simulink model "EScooter_Physical_Architecture"  (R2025b)
settings: Solver=VariableStepAuto  StartTime=0.0  StopTime=10.0  RelTol=1e-3
settings Model: DataDictionary=EScooter_Interfaces.sldd  Creator=louis  LastModifiedBy=louis

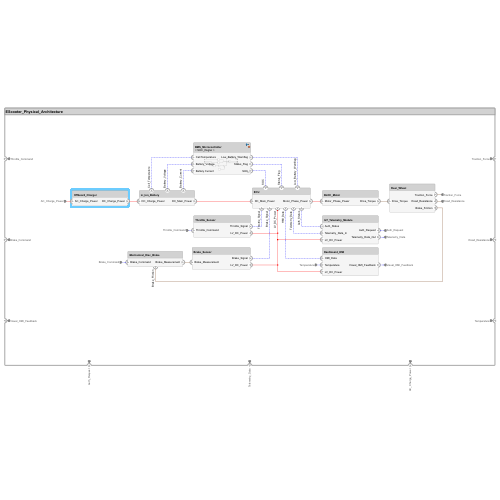
[thumbnail: Simulink's stored preview of the top-level diagram]
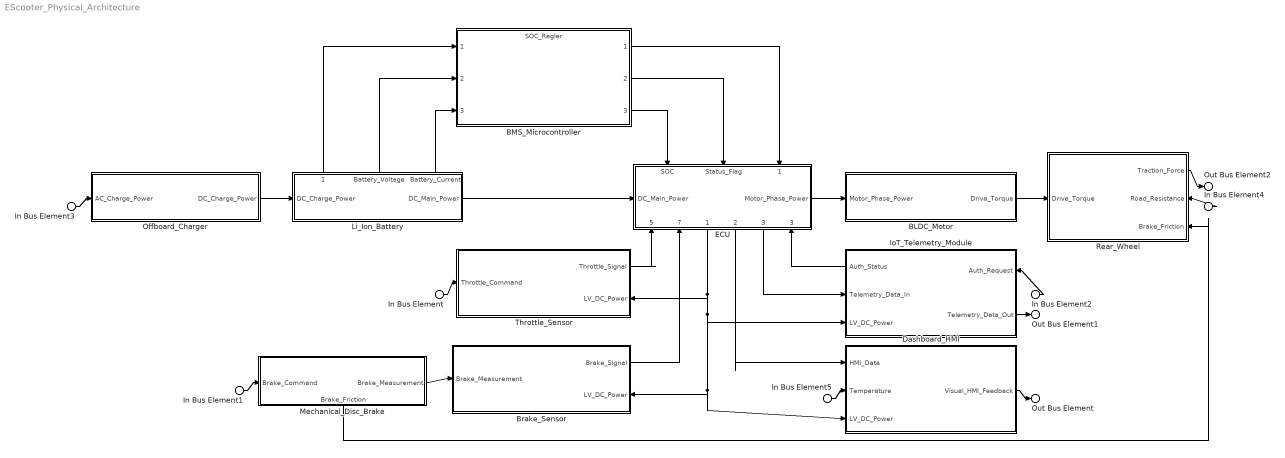
== system EScooter_Physical_Architecture ==
  In Bus Element : Inport  PortName=Throttle_Command
  In Bus Element1 : Inport  Port=2  PortName=Brake_Command
  In Bus Element2 : Inport  Port=3  PortName=Auth_Request
  In Bus Element3 : Inport  Port=4  PortName=AC_Charge_Power
  In Bus Element4 : Inport  Port=5  PortName=Road_Resistance
  In Bus Element5 : Inport  Port=6  PortName=Temperature
  BLDC_Motor : Subsystem
      settings: PortSchema="{\"entries\":[{\"content\":{\"headerSize\":26,\"margin\":15,\"minimumSpacing\":25,\"sides\":[{\"content\":{\"connectorIds\":[\"In1\"]},\"type\":\"ConnectorPlacement.EquallySpacedRectSide\",\"uuid\":\"c7864b0c-a654-4b38-88ce-65a12de73bec\"},{\"content\":{\"connectorIds\":[\"Out1\"],\"side\":\"RIGHT\"},\"type\":\"ConnectorPlacement.EquallySpacedRectSide\",\"uuid\":\"f08a465c-4605-4a04-9f25-0a3dbd0c3078\"},{\"content\":{\"side\":\"TOP\"},\"type\":\"ConnectorPlacement.EquallySpacedRectSide\",\"uuid\":\"8b4ebbb3-fc9a-4287-84ca-4c06f50a2e15\"}]},\"type\":\"ConnectorPlacement.EquallySpacedConnector\",\"uuid\":\"9d8a7b34-6d5f-451a-9c3e-baff170e8406\"}],\"packageUris\":[\"http://schema.mathworks.com/mf0/Connector/R2020b\"],\"version\":\"1.0\"}"
  BMS_Microcontroller : ModelReference  ModelNameDialog=SOC_Regler.slx  SimulationMode=Normal  ModelReferenceVersion=1.3
      settings: PortSchema="{\"entries\":[{\"content\":{\"headerSize\":38,\"margin\":15,\"minimumSpacing\":25,\"sides\":[{\"content\":{\"connectorIds\":[\"In1\",\"In2\",\"In3\"]},\"type\":\"ConnectorPlacement.EquallySpacedRectSide\",\"uuid\":\"4099fe1e-d8ea-4288-98e3-31b6343239af\"},{\"content\":{\"connectorIds\":[\"Out1\",\"Out2\",\"Out3\"],\"side\":\"RIGHT\"},\"type\":\"ConnectorPlacement.EquallySpacedRectSide\",\"uuid\":\"504c5db9-a45d-4379-96ce-ee806ba1f3a5\"},{\"content\":{\"side\":\"TOP\"},\"type\":\"ConnectorPlacement.EquallySpacedRectSide\",\"uuid\":\"29d2f34e-5430-431f-8925-f215a165c8d4\"}]},\"type\":\"ConnectorPlacement.EquallySpacedConnector\",\"uuid\":\"717a3a0c-5e38-4178-bc7e-8ddaf7311f91\"}],\"packageUris\":[\"http://schema.mathworks.com/mf0/Connector/R2020b\"],\"version\":\"1.0\"}"
  Brake_Sensor : Subsystem
      settings: PortSchema="{\"entries\":[{\"content\":{\"headerSize\":26,\"margin\":15,\"minimumSpacing\":25,\"sides\":[{\"content\":{\"connectorIds\":[\"In2\"]},\"type\":\"ConnectorPlacement.EquallySpacedRectSide\",\"uuid\":\"c7864b0c-a654-4b38-88ce-65a12de73bec\"},{\"content\":{\"connectorIds\":[\"Out1\",\"In1\"],\"side\":\"RIGHT\"},\"type\":\"ConnectorPlacement.EquallySpacedRectSide\",\"uuid\":\"f08a465c-4605-4a04-9f25-0a3dbd0c3078\"},{\"content\":{\"side\":\"TOP\"},\"type\":\"ConnectorPlacement.EquallySpacedRectSide\",\"uuid\":\"8b4ebbb3-fc9a-4287-84ca-4c06f50a2e15\"},{\"content\":{\"side\":\"BOTTOM\"},\"type\":\"ConnectorPlacement.EquallySpacedRectSide\",\"uuid\":\"60d35069-caa0-4e85-8360-19172966eb62\"}]},\"type\":\"ConnectorPlacement.EquallySpacedConnector\",\"uuid\":\"9d8a7b34-6d5f-451a-9c3e-baff170e8406\"}],\"packageUris\":[\"http://schema.mathworks.com/mf0/Connector/R2020b\"],\"version\":\"1.0\"}"
  Dashboard_HMI : Subsystem
      settings: PortSchema="{\"entries\":[{\"content\":{\"headerSize\":26,\"margin\":15,\"minimumSpacing\":25,\"sides\":[{\"content\":{\"connectorIds\":[\"In1\",\"In2\",\"In3\"]},\"type\":\"ConnectorPlacement.EquallySpacedRectSide\",\"uuid\":\"c7864b0c-a654-4b38-88ce-65a12de73bec\"},{\"content\":{\"connectorIds\":[\"Out1\"],\"side\":\"RIGHT\"},\"type\":\"ConnectorPlacement.EquallySpacedRectSide\",\"uuid\":\"f08a465c-4605-4a04-9f25-0a3dbd0c3078\"},{\"content\":{\"side\":\"TOP\"},\"type\":\"ConnectorPlacement.EquallySpacedRectSide\",\"uuid\":\"8b4ebbb3-fc9a-4287-84ca-4c06f50a2e15\"}]},\"type\":\"ConnectorPlacement.EquallySpacedConnector\",\"uuid\":\"9d8a7b34-6d5f-451a-9c3e-baff170e8406\"}],\"packageUris\":[\"http://schema.mathworks.com/mf0/Connector/R2020b\"],\"version\":\"1.0\"}"
  ECU : Subsystem
      settings: PortSchema="{\"entries\":[{\"content\":{\"headerSize\":26,\"margin\":15,\"minimumSpacing\":25,\"sides\":[{\"content\":{\"connectorIds\":[\"In6\"]},\"type\":\"ConnectorPlacement.EquallySpacedRectSide\",\"uuid\":\"c7864b0c-a654-4b38-88ce-65a12de73bec\"},{\"content\":{\"connectorIds\":[\"Out4\"],\"side\":\"RIGHT\"},\"type\":\"ConnectorPlacement.EquallySpacedRectSide\",\"uuid\":\"f08a465c-4605-4a04-9f25-0a3dbd0c3078\"},{\"content\":{\"connectorIds\":[\"In2\",\"In4\",\"In1\"],\"side\":\"TOP\"},\"type\":\"ConnectorPlacement.EquallySpacedRectSide\",\"uuid\":\"8b4ebbb3-fc9a-4287-84ca-4c06f50a2e15\"},{\"content\":{\"connectorIds\":[\"In5\",\"In7\",\"Out1\",\"Out2\",\"Out3\",\"In3\"],\"side\":\"BOTTOM\"},\"type\":\"ConnectorPlacement.EquallySpacedRectSide\",\"uuid\":\"c8544b79-1559-4f8f-8e3a-48f86e4e49c0\"}]},\"type\":\"ConnectorPlacement.EquallySpacedConnector\",\"uuid\":\"9d8a7b34-6d5f-451a-9c3e-baff170e8406\"}],\"packageUris\":[\"http://schema.mathworks.com/mf0/Connector/R2020b\"],\"version\":\"1.0\"}"
  IoT_Telemetry_Module : Subsystem
      settings: PortSchema="{\"entries\":[{\"content\":{\"headerSize\":26,\"margin\":15,\"minimumSpacing\":25,\"sides\":[{\"content\":{\"connectorIds\":[\"Out1\",\"In3\",\"In2\"]},\"type\":\"ConnectorPlacement.EquallySpacedRectSide\",\"uuid\":\"c7864b0c-a654-4b38-88ce-65a12de73bec\"},{\"content\":{\"connectorIds\":[\"In1\",\"Out2\"],\"side\":\"RIGHT\"},\"type\":\"ConnectorPlacement.EquallySpacedRectSide\",\"uuid\":\"f08a465c-4605-4a04-9f25-0a3dbd0c3078\"},{\"content\":{\"side\":\"TOP\"},\"type\":\"ConnectorPlacement.EquallySpacedRectSide\",\"uuid\":\"8b4ebbb3-fc9a-4287-84ca-4c06f50a2e15\"},{\"content\":{\"side\":\"BOTTOM\"},\"type\":\"ConnectorPlacement.EquallySpacedRectSide\",\"uuid\":\"026f311c-75bd-495b-b3f1-5519b50e0082\"}]},\"type\":\"ConnectorPlacement.EquallySpacedConnector\",\"uuid\":\"9d8a7b34-6d5f-451a-9c3e-baff170e8406\"}],\"packageUris\":[\"http://schema.mathworks.com/mf0/Connector/R2020b\"],\"version\":\"1.0\"}"
  Li_Ion_Battery : Subsystem
      settings: PortSchema="{\"entries\":[{\"content\":{\"headerSize\":26,\"margin\":15,\"minimumSpacing\":25,\"sides\":[{\"content\":{\"connectorIds\":[\"In1\"]},\"type\":\"ConnectorPlacement.EquallySpacedRectSide\",\"uuid\":\"c7864b0c-a654-4b38-88ce-65a12de73bec\"},{\"content\":{\"connectorIds\":[\"Out4\"],\"side\":\"RIGHT\"},\"type\":\"ConnectorPlacement.EquallySpacedRectSide\",\"uuid\":\"f08a465c-4605-4a04-9f25-0a3dbd0c3078\"},{\"content\":{\"connectorIds\":[\"Out1\",\"Out2\",\"Out3\"],\"side\":\"TOP\"},\"type\":\"ConnectorPlacement.EquallySpacedRectSide\",\"uuid\":\"8b4ebbb3-fc9a-4287-84ca-4c06f50a2e15\"},{\"content\":{\"side\":\"BOTTOM\"},\"type\":\"ConnectorPlacement.EquallySpacedRectSide\",\"uuid\":\"a12c9fad-78c1-47b3-951e-87e8443312d3\"}]},\"type\":\"ConnectorPlacement.EquallySpacedConnector\",\"uuid\":\"9d8a7b34-6d5f-451a-9c3e-baff170e8406\"}],\"packageUris\":[\"http://schema.mathworks.com/mf0/Connector/R2020b\"],\"version\":\"1.0\"}"
  Mechanical_Disc_Brake : Subsystem
      settings: PortSchema="{\"entries\":[{\"content\":{\"headerSize\":26,\"margin\":15,\"minimumSpacing\":25,\"sides\":[{\"content\":{\"connectorIds\":[\"In1\"]},\"type\":\"ConnectorPlacement.EquallySpacedRectSide\",\"uuid\":\"c0a0fd83-8e6b-4996-80ba-c62bfd1e5bac\"},{\"content\":{\"connectorIds\":[\"Out1\"],\"side\":\"RIGHT\"},\"type\":\"ConnectorPlacement.EquallySpacedRectSide\",\"uuid\":\"b459cc4e-9c94-4f14-9d9c-94419e22855a\"},{\"content\":{\"side\":\"TOP\"},\"type\":\"ConnectorPlacement.EquallySpacedRectSide\",\"uuid\":\"d2d10086-fe87-4682-8840-902f46fdf630\"},{\"content\":{\"connectorIds\":[\"Out2\"],\"side\":\"BOTTOM\"},\"type\":\"ConnectorPlacement.EquallySpacedRectSide\",\"uuid\":\"3ddfbb52-bdc8-43fc-9731-c09ce9f1a202\"}]},\"type\":\"ConnectorPlacement.EquallySpacedConnector\",\"uuid\":\"74f202a8-1c68-49b4-8447-64ee5fb276eb\"}],\"packageUris\":[\"http://schema.mathworks.com/mf0/Connector/R2020b\"],\"version\":\"1.0\"}"
  Offboard_Charger : Subsystem  Description=Ladeleistung 350W (Ausgeklammert aus SWaP, da nur im Charging-State aktiv)
      settings: PortSchema="{\"entries\":[{\"content\":{\"headerSize\":26,\"margin\":15,\"minimumSpacing\":25,\"sides\":[{\"content\":{\"connectorIds\":[\"In1\"]},\"type\":\"ConnectorPlacement.EquallySpacedRectSide\",\"uuid\":\"c0a0fd83-8e6b-4996-80ba-c62bfd1e5bac\"},{\"content\":{\"connectorIds\":[\"Out1\"],\"side\":\"RIGHT\"},\"type\":\"ConnectorPlacement.EquallySpacedRectSide\",\"uuid\":\"b459cc4e-9c94-4f14-9d9c-94419e22855a\"},{\"content\":{\"side\":\"TOP\"},\"type\":\"ConnectorPlacement.EquallySpacedRectSide\",\"uuid\":\"d2d10086-fe87-4682-8840-902f46fdf630\"}]},\"type\":\"ConnectorPlacement.EquallySpacedConnector\",\"uuid\":\"74f202a8-1c68-49b4-8447-64ee5fb276eb\"}],\"packageUris\":[\"http://schema.mathworks.com/mf0/Connector/R2020b\"],\"version\":\"1.0\"}"
  Rear_Wheel : Subsystem
      settings: PortSchema="{\"entries\":[{\"content\":{\"headerSize\":26,\"margin\":15,\"minimumSpacing\":25,\"sides\":[{\"content\":{\"connectorIds\":[\"In3\"]},\"type\":\"ConnectorPlacement.EquallySpacedRectSide\",\"uuid\":\"c7864b0c-a654-4b38-88ce-65a12de73bec\"},{\"content\":{\"connectorIds\":[\"Out1\",\"In1\",\"In2\"],\"side\":\"RIGHT\"},\"type\":\"ConnectorPlacement.EquallySpacedRectSide\",\"uuid\":\"f08a465c-4605-4a04-9f25-0a3dbd0c3078\"},{\"content\":{\"side\":\"TOP\"},\"type\":\"ConnectorPlacement.EquallySpacedRectSide\",\"uuid\":\"8b4ebbb3-fc9a-4287-84ca-4c06f50a2e15\"}]},\"type\":\"ConnectorPlacement.EquallySpacedConnector\",\"uuid\":\"9d8a7b34-6d5f-451a-9c3e-baff170e8406\"}],\"packageUris\":[\"http://schema.mathworks.com/mf0/Connector/R2020b\"],\"version\":\"1.0\"}"
  Throttle_Sensor : Subsystem
      settings: PortSchema="{\"entries\":[{\"content\":{\"headerSize\":26,\"margin\":15,\"minimumSpacing\":25,\"sides\":[{\"content\":{\"connectorIds\":[\"In2\"]},\"type\":\"ConnectorPlacement.EquallySpacedRectSide\",\"uuid\":\"c7864b0c-a654-4b38-88ce-65a12de73bec\"},{\"content\":{\"connectorIds\":[\"Out1\",\"In1\"],\"side\":\"RIGHT\"},\"type\":\"ConnectorPlacement.EquallySpacedRectSide\",\"uuid\":\"f08a465c-4605-4a04-9f25-0a3dbd0c3078\"},{\"content\":{\"side\":\"TOP\"},\"type\":\"ConnectorPlacement.EquallySpacedRectSide\",\"uuid\":\"8b4ebbb3-fc9a-4287-84ca-4c06f50a2e15\"}]},\"type\":\"ConnectorPlacement.EquallySpacedConnector\",\"uuid\":\"9d8a7b34-6d5f-451a-9c3e-baff170e8406\"}],\"packageUris\":[\"http://schema.mathworks.com/mf0/Connector/R2020b\"],\"version\":\"1.0\"}"
  Out Bus Element : Outport  PortName=Visual_HMI_Feedback
  Out Bus Element1 : Outport  Port=2  PortName=Telemetry_Data
  Out Bus Element2 : Outport  Port=3  PortName=Traction_Force
  wires:
  Li_Ion_Battery/4(DC_Main_Power) -> ECU/6(DC_Main_Power)
  Throttle_Sensor/1(Throttle_Signal) -> ECU/5(Throttle_Signal)
  ECU/3(Telemetry_Data) -> IoT_Telemetry_Module/3(Telemetry_Data_In)
  BLDC_Motor/1(Drive_Torque) -> Rear_Wheel/3(Drive_Torque)
  ECU/2(HMI_Data) -> Dashboard_HMI/1(HMI_Data)
  ECU/4(Motor_Phase_Power) -> BLDC_Motor/1(Motor_Phase_Power)
  Li_Ion_Battery/2(Battery_Voltage) -> BMS_Microcontroller/2
  BMS_Microcontroller/1 -> ECU/1(Low_Battery_Warnflag)
  BMS_Microcontroller/2 -> ECU/4(Status_Flag)
  BMS_Microcontroller/3 -> ECU/2(SOC)
  Offboard_Charger/1(DC_Charge_Power) -> Li_Ion_Battery/1(DC_Charge_Power)
  In Bus Element/1 -> Throttle_Sensor/2(Throttle_Command)
  In Bus Element3/1 -> Offboard_Charger/1(AC_Charge_Power)
  In Bus Element5/1 -> Dashboard_HMI/2(Temperature)
  Dashboard_HMI/1(Visual_HMI_Feedback) -> Out Bus Element/1
  IoT_Telemetry_Module/2(Telemetry_Data_Out) -> Out Bus Element1/1
  In Bus Element4/1 -> Rear_Wheel/1(Road_Resistance)
  Rear_Wheel/1(Traction_Force) -> Out Bus Element2/1
  Mechanical_Disc_Brake/2(Brake_Friction) -> Rear_Wheel/2(Brake_Friction)
  Mechanical_Disc_Brake/1(Brake_Measurement) -> Brake_Sensor/2(Brake_Measurement)
  In Bus Element1/1 -> Mechanical_Disc_Brake/1(Brake_Command)
  Brake_Sensor/1(Brake_Signal) -> ECU/7(Brake_Signal)
  In Bus Element2/1 -> IoT_Telemetry_Module/1(Auth_Request)
  IoT_Telemetry_Module/1(Auth_Status) -> ECU/3(Auth_Status)
  ECU/1(LV_DC_Power) -> IoT_Telemetry_Module/2(LV_DC_Power), Dashboard_HMI/3(LV_DC_Power), Brake_Sensor/1(LV_DC_Power), Throttle_Sensor/1(LV_DC_Power)
  Li_Ion_Battery/3(Battery_Current) -> BMS_Microcontroller/3
  Li_Ion_Battery/1(Cell_Temperature) -> BMS_Microcontroller/1

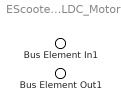
== system EScooter_Physical_Architecture/BLDC_Motor ==
  Bus Element In1 : Inport  PortName=Motor_Phase_Power
  Bus Element Out1 : Outport  PortName=Drive_Torque

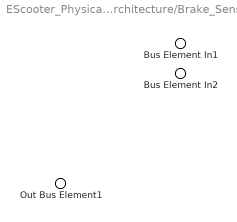
== system EScooter_Physical_Architecture/Brake_Sensor ==
  Bus Element In2 : Inport  PortName=LV_DC_Power
  Bus Element In1 : Inport  Port=2  PortName=Brake_Measurement
  Out Bus Element1 : Outport  PortName=Brake_Signal

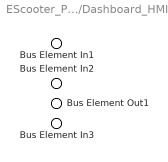
== system EScooter_Physical_Architecture/Dashboard_HMI ==
  Bus Element In1 : Inport  PortName=HMI_Data
  Bus Element In2 : Inport  Port=2  PortName=Temperature
  Bus Element In3 : Inport  Port=3  PortName=LV_DC_Power
  Bus Element Out1 : Outport  PortName=Visual_HMI_Feedback

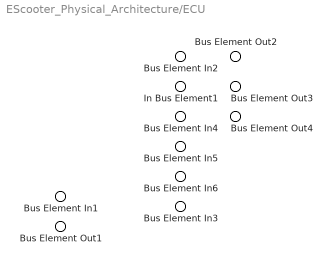
== system EScooter_Physical_Architecture/ECU ==
  Bus Element In4 : Inport  PortName=Low_Battery_Warnflag
  Bus Element In6 : Inport  Port=2  PortName=SOC
  Bus Element In3 : Inport  Port=3  PortName=Auth_Status
  Bus Element In5 : Inport  Port=4  PortName=Status_Flag
  Bus Element In2 : Inport  Port=5  PortName=Throttle_Signal
  Bus Element In1 : Inport  Port=6  PortName=DC_Main_Power
  In Bus Element1 : Inport  Port=7  PortName=Brake_Signal
  Bus Element Out4 : Outport  PortName=LV_DC_Power
  Bus Element Out3 : Outport  Port=2  PortName=HMI_Data
  Bus Element Out2 : Outport  Port=3  PortName=Telemetry_Data
  Bus Element Out1 : Outport  Port=4  PortName=Motor_Phase_Power

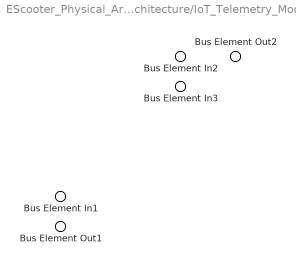
== system EScooter_Physical_Architecture/IoT_Telemetry_Module ==
  Bus Element In2 : Inport  PortName=Auth_Request
  Bus Element In3 : Inport  Port=2  PortName=LV_DC_Power
  Bus Element In1 : Inport  Port=3  PortName=Telemetry_Data_In
  Bus Element Out2 : Outport  PortName=Auth_Status
  Bus Element Out1 : Outport  Port=2  PortName=Telemetry_Data_Out

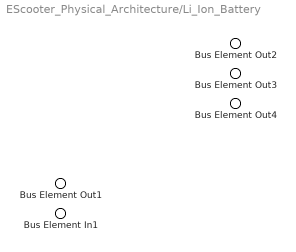
== system EScooter_Physical_Architecture/Li_Ion_Battery ==
  Bus Element In1 : Inport  PortName=DC_Charge_Power
  Bus Element Out2 : Outport  PortName=Cell_Temperature
  Bus Element Out3 : Outport  Port=2  PortName=Battery_Voltage
  Bus Element Out4 : Outport  Port=3  PortName=Battery_Current
  Bus Element Out1 : Outport  Port=4  PortName=DC_Main_Power

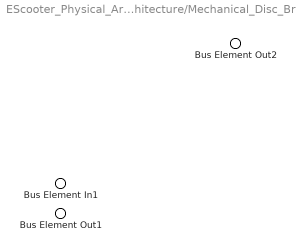
== system EScooter_Physical_Architecture/Mechanical_Disc_Brake ==
  Bus Element In1 : Inport  PortName=Brake_Command
  Bus Element Out2 : Outport  PortName=Brake_Measurement
  Bus Element Out1 : Outport  Port=2  PortName=Brake_Friction

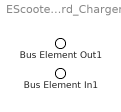
== system EScooter_Physical_Architecture/Offboard_Charger ==
  Bus Element In1 : Inport  PortName=AC_Charge_Power
  Bus Element Out1 : Outport  PortName=DC_Charge_Power

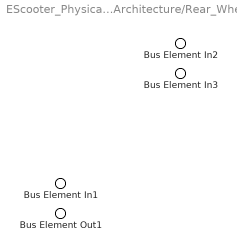
== system EScooter_Physical_Architecture/Rear_Wheel ==
  Bus Element In2 : Inport  PortName=Road_Resistance
  Bus Element In3 : Inport  Port=2  PortName=Brake_Friction
  Bus Element In1 : Inport  Port=3  PortName=Drive_Torque
  Bus Element Out1 : Outport  PortName=Traction_Force

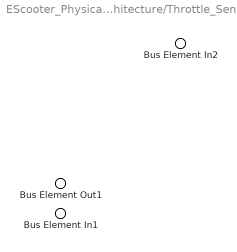
== system EScooter_Physical_Architecture/Throttle_Sensor ==
  Bus Element In2 : Inport  PortName=LV_DC_Power
  Bus Element In1 : Inport  Port=2  PortName=Throttle_Command
  Bus Element Out1 : Outport  PortName=Throttle_Signal
